simulink model "dimensions_equivalent"  (R2021b)
settings: Solver=VariableStepAuto  StartTime=0.0  StopTime=10.0  RelTol=1e-3
undefined symbols (not defined in the file): DiscIntNeverNeededParam, magnitude, Newton, Raphson
libraries: simulink x80, slpidlib x2
(part 1 of 3)
settings Model: Creator=user  LastModifiedBy=cemery
settings SolverCC: AlgebraicLoopSolver=TrustRegion
settings DataIOCC: ReturnWorkspaceOutputs=off
settings DebuggingCC: SFMachineParentedDataDiag=warning  ArithmeticOperatorsInVariantConditions=warning
settings SFSimCC: SimUseLocalCustomCode=off  CustomCodeUndefinedFunction=UseInterfaceOnly
settings RTWCC: RTWUseLocalCustomCode=off

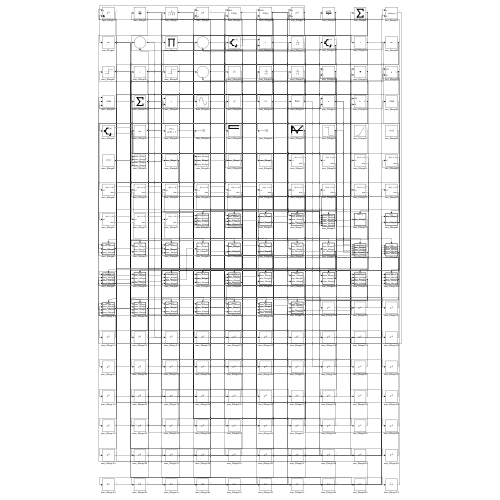
[thumbnail: Simulink's stored preview of the top-level diagram]
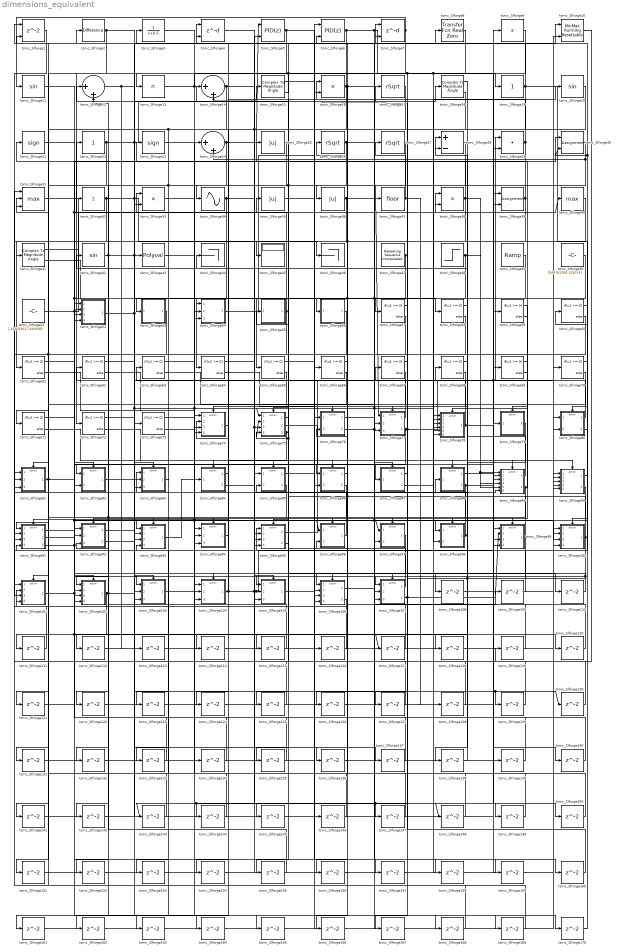
== system dimensions_equivalent ==
  tsmc_Slforge1 : Delay  ShowEnablePort=on  SampleTime=1
      settings: InputPortMap=u0,e6
  tsmc_Slforge10 : simulink/Math Operations/MinMax Running Resettable  Function=min  vinit=0.0
  tsmc_Slforge100 : Subsystem  TreatAsAtomicUnit=on
  tsmc_Slforge101 : Subsystem  TreatAsAtomicUnit=on
  tsmc_Slforge102 : Subsystem  TreatAsAtomicUnit=on
  tsmc_Slforge103 : Subsystem  TreatAsAtomicUnit=on
  tsmc_Slforge104 : Subsystem  TreatAsAtomicUnit=on
  tsmc_Slforge105 : Subsystem  TreatAsAtomicUnit=on
  tsmc_Slforge106 : Subsystem  TreatAsAtomicUnit=on
  tsmc_Slforge107 : Subsystem  TreatAsAtomicUnit=on
  tsmc_Slforge{108..170} (63 alike) : Delay  SampleTime=1
  tsmc_Slforge11 : Trigonometry
  tsmc_Slforge12 : Sum  Inputs=|++
  tsmc_Slforge13 : Product  Inputs=*
  tsmc_Slforge14 : Sum  Inputs=|++
  tsmc_Slforge15 : ComplexToMagnitudeAngle
  tsmc_Slforge16 : Product  Inputs=**
  tsmc_Slforge17 : Sqrt  Operator=rSqrt  AlgorithmType=Newton-Raphson  SaturateOnIntegerOverflow=on
  tsmc_Slforge18 : ComplexToMagnitudeAngle
  tsmc_Slforge19 : simulink/Math Operations/Slider Gain  gain=1  low=0  high=2
  tsmc_Slforge2 : simulink/Discrete/Difference  ICPrevInput=0.0  OutMin=[]  OutMax=[]  OutDataTypeStr=Inherit: Inherit via back propagation  OutDataType=fixdt(1, 16)  OutScaling=2^-10  DoSatur=off
  tsmc_Slforge20 : Trigonometry
  tsmc_Slforge21 : Signum
  tsmc_Slforge22 : simulink/Math Operations/Slider Gain  gain=1  low=0  high=2
  tsmc_Slforge23 : Signum
  tsmc_Slforge24 : Sum  Inputs=|++
  tsmc_Slforge25 : Abs
  tsmc_Slforge26 : Sqrt  Operator=rSqrt  AlgorithmType=Newton-Raphson  SaturateOnIntegerOverflow=on
  tsmc_Slforge27 : Sqrt  Operator=rSqrt  AlgorithmType=Newton-Raphson  SaturateOnIntegerOverflow=on
  tsmc_Slforge28 : Sum  Inputs=+-
  tsmc_Slforge29 : DotProduct  InputSameDT=on  OutDataTypeStr=Inherit: Inherit via internal rule
  tsmc_Slforge3 : DiscreteTransferFcn  SampleTime=1
  tsmc_Slforge30 : Assignment  DiagnosticForDimensions=Warning  IndexOptions=Index vector (dialog)  Indices=1  OutputSizes=1
  tsmc_Slforge31 : MinMax  Function=max  Inputs=3
  tsmc_Slforge32 : Sum  Inputs=+
  tsmc_Slforge33 : Product  Inputs=**
  tsmc_Slforge34 : Sin  TimeSource=Use external signal  SampleTime=0
  tsmc_Slforge35 : Abs
  tsmc_Slforge36 : Abs
  tsmc_Slforge37 : Rounding
  tsmc_Slforge38 : Product
  tsmc_Slforge39 : Assignment  DiagnosticForDimensions=Warning  IndexOptions=Index vector (dialog)  Indices=1  OutputSizes=1
  tsmc_Slforge4 : Delay  DelayLengthSource=Input port  SampleTime=1
      settings: InputPortMap=u0,p1
  tsmc_Slforge40 : MinMax  Function=max
  tsmc_Slforge41 : ComplexToMagnitudeAngle
  tsmc_Slforge42 : Trigonometry
  tsmc_Slforge43 : Polyval  Coefs=[ +2.081618890e-019, -1.441693666e-014, +4.719686976e-010, -8.536869453e-006, +1.621573104e-001, -8.087801117e+001 ]
  tsmc_Slforge44 : Terminator
  tsmc_Slforge45 : Display
  tsmc_Slforge46 : Terminator
  tsmc_Slforge47 : simulink/Sources/Repeating Sequence Interpolated  OutValues=[-224844362.242719, 761907502.904714, -469417062.555968, 95128126.771430, 892289046.180384]  TimeValues=[0 0.1 0.5 0.6 1].'  LookUpMeth=Use Input Below  tsamp=0.01  OutMin=[]  OutMax=[]  OutDataTypeStr=double  OutputDataTypeScalingMode=double  OutDataType=fixdt(0,8)  OutScaling=2^-10
  tsmc_Slforge48 : Step  Time=[25.000000]  Before=[335295422.757427]  After=[-716731590.646786]  SampleTime=0
  tsmc_Slforge49 : simulink/Sources/Ramp  slope=[-2914.888673]  start=[19.513339]  InitialOutput=[436099.857088]
  tsmc_Slforge5 : slpidlib/PID Controller (2DOF)  Controller=PID  Form=Parallel  TimeDomain=Discrete-time  UseExternalTs=off  SampleTime=1  IntegratorMethod=Forward Euler  FilterMethod=Forward Euler  ControllerParametersSource=internal  P=1  I=1  D=0  UseFilter=on  N=100  b=1  c=1  TunerSelectOption=Transfer Function Based (PID Tuner App)  InitialConditionSource=internal  InitialConditionForIntegrator=0  InitialConditionForFilter=0  DifferentiatorICPrevScaledInput=0  ExternalReset=none  TrackingMode=off  Kt=1  LimitOutput=off  SatLimitsSource=internal  UpperSaturationLimit=inf  LowerSaturationLimit=-inf  LinearizeAsGain=off  AntiWindupMode=none  Kb=1  POutMin=[]  POutMax=[]  IOutMin=[]  IOutMax=[]  DOutMin=[]  DOutMax=[]  NOutMin=[]  NOutMax=[]  bOutMin=[]  bOutMax=[]  cOutMin=[]  cOutMax=[]  SumOutMin=[]  SumOutMax=[]  SaturationOutMin=[]  SaturationOutMax=[]  PParamMin=[]  PParamMax=[]  IParamMin=[]  IParamMax=[]  DParamMin=[]  DParamMax=[]  NParamMin=[]  NParamMax=[]  bParamMin=[]  bParamMax=[]  cParamMin=[]  cParamMax=[]  KbParamMin=[]  KbParamMax=[]  KtParamMin=[]  KtParamMax=[]  KbOutMin=[]  KbOutMax=[]  KtOutMin=[]  KtOutMax=[]  IntegratorOutMin=[]  IntegratorOutMax=[]  FilterOutMin=[]  FilterOutMax=[]  SumI1OutMin=[]  SumI1OutMax=[]  SumI2OutMin=[]  SumI2OutMax=[]  SumI3OutMin=[]  SumI3OutMax=[]  SumI4OutMin=[]  SumI4OutMax=[]  SumDOutMin=[]  SumDOutMax=[]  Sum1OutMin=[]  Sum1OutMax=[]  Sum2OutMin=[]  Sum2OutMax=[]  Sum3OutMin=[]  Sum3OutMax=[]  DifferentiatorOutMin=[]  DifferentiatorOutMax=[]  FilterDiffOutCoefMin=[]  FilterDiffOutCoefMax=[]  ReciprocalOutMin=[]  ReciprocalOutMax=[]  SumDenOutMin=[]  SumDenOutMax=[]  SumNumOutMin=[]  SumNumOutMax=[]  DivideOutMin=[]  DivideOutMax=[]  UdiffTsProdOutMin=[]  UdiffTsProdOutMax=[]  NTsProdOutMin=[]  NTsProdOutMax=[]  UintegralTsProdOutMin=[]  UintegralTsProdOutMax=[]  UngainTsProdOutMin=[]  UngainTsProdOutMax=[]  IntegratorContinuousStateAttributes=''  IntegratorStateMustResolveToSignalObject=off  IntegratorRTWStateStorageClass=Auto  FilterContinuousStateAttributes=''  FilterStateMustResolveToSignalObject=off  FilterRTWStateStorageClass=Auto  ParallelPVariant=InternalParameters  IdealPVariant=Disabled  IVariant=InternalParameters  DVariant=InternalParameters  bVariant=InternalParameters  cVariant=InternalParameters  IntegratorVariant=Discrete  SatVariant=Disabled  AWVariant=Passthrough  PCopyVariant=Disabled  TRVariant=Disabled  FdbkBlocksVariant=Forward  IdealPFdbkVariant=Disabled  SatFdbkVariant=Disabled  DerivativeFilterVariant=ForwardEulerFilter  NVariant=InternalParameters  NCopyVariant=Disabled  FilterICVariant=InternalICsFilter  IntegratorICVariant=InternalICs  ExternalResetVariant=Disabled  TRSumVariant=Passthrough  SumFdbkVariant=Disabled  SumVariant=Sum_PID  TsampFilterVariant=InternalTs  TsampNgainVariant=Passthrough  TsampIntegralVariant=Passthrough  ExternalSaturationOutDataTypeStr=Inherit: Same as second input
      settings: SourceProductBaseCode=SL
  tsmc_Slforge50 : Constant  Value=[844181906.319014]  SampleTime=1
  tsmc_Slforge51 : Constant  Value=[-323053627.840698]  SampleTime=1
  tsmc_Slforge52 : Subsystem
  tsmc_Slforge53 : Subsystem
  tsmc_Slforge54 : Subsystem
  tsmc_Slforge55 : Subsystem
  tsmc_Slforge56 : Subsystem
  tsmc_Slforge{57..73} (17 alike) : If  IfExpression=u1 >= 0  SampleTime=1
  tsmc_Slforge6 : slpidlib/PID Controller (2DOF)  Controller=PID  Form=Parallel  TimeDomain=Discrete-time  UseExternalTs=off  SampleTime=1  IntegratorMethod=Forward Euler  FilterMethod=Forward Euler  ControllerParametersSource=internal  P=1  I=1  D=0  UseFilter=on  N=100  b=1  c=1  TunerSelectOption=Transfer Function Based (PID Tuner App)  InitialConditionSource=internal  InitialConditionForIntegrator=0  InitialConditionForFilter=0  DifferentiatorICPrevScaledInput=0  ExternalReset=none  TrackingMode=off  Kt=1  LimitOutput=off  SatLimitsSource=internal  UpperSaturationLimit=inf  LowerSaturationLimit=-inf  LinearizeAsGain=off  AntiWindupMode=none  Kb=1  POutMin=[]  POutMax=[]  IOutMin=[]  IOutMax=[]  DOutMin=[]  DOutMax=[]  NOutMin=[]  NOutMax=[]  bOutMin=[]  bOutMax=[]  cOutMin=[]  cOutMax=[]  SumOutMin=[]  SumOutMax=[]  SaturationOutMin=[]  SaturationOutMax=[]  PParamMin=[]  PParamMax=[]  IParamMin=[]  IParamMax=[]  DParamMin=[]  DParamMax=[]  NParamMin=[]  NParamMax=[]  bParamMin=[]  bParamMax=[]  cParamMin=[]  cParamMax=[]  KbParamMin=[]  KbParamMax=[]  KtParamMin=[]  KtParamMax=[]  KbOutMin=[]  KbOutMax=[]  KtOutMin=[]  KtOutMax=[]  IntegratorOutMin=[]  IntegratorOutMax=[]  FilterOutMin=[]  FilterOutMax=[]  SumI1OutMin=[]  SumI1OutMax=[]  SumI2OutMin=[]  SumI2OutMax=[]  SumI3OutMin=[]  SumI3OutMax=[]  SumI4OutMin=[]  SumI4OutMax=[]  SumDOutMin=[]  SumDOutMax=[]  Sum1OutMin=[]  Sum1OutMax=[]  Sum2OutMin=[]  Sum2OutMax=[]  Sum3OutMin=[]  Sum3OutMax=[]  DifferentiatorOutMin=[]  DifferentiatorOutMax=[]  FilterDiffOutCoefMin=[]  FilterDiffOutCoefMax=[]  ReciprocalOutMin=[]  ReciprocalOutMax=[]  SumDenOutMin=[]  SumDenOutMax=[]  SumNumOutMin=[]  SumNumOutMax=[]  DivideOutMin=[]  DivideOutMax=[]  UdiffTsProdOutMin=[]  UdiffTsProdOutMax=[]  NTsProdOutMin=[]  NTsProdOutMax=[]  UintegralTsProdOutMin=[]  UintegralTsProdOutMax=[]  UngainTsProdOutMin=[]  UngainTsProdOutMax=[]  IntegratorContinuousStateAttributes=''  IntegratorStateMustResolveToSignalObject=off  IntegratorRTWStateStorageClass=Auto  FilterContinuousStateAttributes=''  FilterStateMustResolveToSignalObject=off  FilterRTWStateStorageClass=Auto  ParallelPVariant=InternalParameters  IdealPVariant=Disabled  IVariant=InternalParameters  DVariant=InternalParameters  bVariant=InternalParameters  cVariant=InternalParameters  IntegratorVariant=Discrete  SatVariant=Disabled  AWVariant=Passthrough  PCopyVariant=Disabled  TRVariant=Disabled  FdbkBlocksVariant=Forward  IdealPFdbkVariant=Disabled  SatFdbkVariant=Disabled  DerivativeFilterVariant=ForwardEulerFilter  NVariant=InternalParameters  NCopyVariant=Disabled  FilterICVariant=InternalICsFilter  IntegratorICVariant=InternalICs  ExternalResetVariant=Disabled  TRSumVariant=Passthrough  SumFdbkVariant=Disabled  SumVariant=Sum_PID  TsampFilterVariant=InternalTs  TsampNgainVariant=Passthrough  TsampIntegralVariant=Passthrough  ExternalSaturationOutDataTypeStr=Inherit: Same as second input
      settings: SourceProductBaseCode=SL
  tsmc_Slforge7 : Delay  DelayLengthSource=Input port  SampleTime=1
      settings: InputPortMap=u0,p1
  tsmc_Slforge74 : Subsystem  TreatAsAtomicUnit=on
  tsmc_Slforge75 : Subsystem  TreatAsAtomicUnit=on
  tsmc_Slforge76 : Subsystem  TreatAsAtomicUnit=on
  tsmc_Slforge77 : Subsystem  TreatAsAtomicUnit=on
  tsmc_Slforge78 : Subsystem  TreatAsAtomicUnit=on
  tsmc_Slforge79 : Subsystem  TreatAsAtomicUnit=on
  tsmc_Slforge8 : simulink/Discrete/Transfer Fcn Real Zero  ZeroZ=0.75  ICPrevInput=0.0  DoSatur=off
      settings: SourceProductBaseCode=SL
  tsmc_Slforge80 : Subsystem  TreatAsAtomicUnit=on
  tsmc_Slforge81 : Subsystem  TreatAsAtomicUnit=on
  tsmc_Slforge82 : Subsystem  TreatAsAtomicUnit=on
  tsmc_Slforge83 : Subsystem  TreatAsAtomicUnit=on
  tsmc_Slforge84 : Subsystem  TreatAsAtomicUnit=on
  tsmc_Slforge85 : Subsystem  TreatAsAtomicUnit=on
  tsmc_Slforge86 : Subsystem  TreatAsAtomicUnit=on
  tsmc_Slforge87 : Subsystem  TreatAsAtomicUnit=on
  tsmc_Slforge88 : Subsystem  TreatAsAtomicUnit=on
  tsmc_Slforge89 : Subsystem  TreatAsAtomicUnit=on
  tsmc_Slforge9 : Sum  Inputs=+
  tsmc_Slforge90 : Subsystem  TreatAsAtomicUnit=on
  tsmc_Slforge91 : Subsystem  TreatAsAtomicUnit=on
  tsmc_Slforge92 : Subsystem  TreatAsAtomicUnit=on
  tsmc_Slforge93 : Subsystem  TreatAsAtomicUnit=on
  tsmc_Slforge94 : Subsystem  TreatAsAtomicUnit=on
  tsmc_Slforge95 : Subsystem  TreatAsAtomicUnit=on
  tsmc_Slforge96 : Subsystem  TreatAsAtomicUnit=on
  tsmc_Slforge97 : Subsystem  TreatAsAtomicUnit=on
  tsmc_Slforge98 : Subsystem  TreatAsAtomicUnit=on
  tsmc_Slforge99 : Subsystem  TreatAsAtomicUnit=on
  wires:
  tsmc_Slforge26/1 -> tsmc_Slforge162/1, tsmc_Slforge163/1, tsmc_Slforge89/3(tsmc_Slforge25)
  tsmc_Slforge95/1(tsmc_Slforge2) -> tsmc_Slforge29/1
  tsmc_Slforge36/1 -> tsmc_Slforge77/1(tsmc_Slforge1), tsmc_Slforge45/1
  tsmc_Slforge102/1(tsmc_Slforge2) -> tsmc_Slforge129/1, tsmc_Slforge130/1, tsmc_Slforge132/1, tsmc_Slforge131/1
  tsmc_Slforge50/1 -> tsmc_Slforge53/1(tsmc_Slforge1)
  tsmc_Slforge49/1 -> tsmc_Slforge64/1
  tsmc_Slforge19/1 -> tsmc_Slforge95/1(tsmc_Slforge1), tsmc_Slforge7/2, tsmc_Slforge95/4(tsmc_Slforge28)
  tsmc_Slforge93/1(tsmc_Slforge2) -> tsmc_Slforge84/1(tsmc_Slforge1)
  tsmc_Slforge39/1 -> tsmc_Slforge102/4(tsmc_Slforge29), tsmc_Slforge156/1, tsmc_Slforge36/1
  tsmc_Slforge2/1 -> tsmc_Slforge95/2(tsmc_Slforge26), tsmc_Slforge78/6(tsmc_Slforge24), tsmc_Slforge72/1
  tsmc_Slforge32/1 -> tsmc_Slforge46/1, tsmc_Slforge169/1, tsmc_Slforge101/3(tsmc_Slforge30)
  tsmc_Slforge3/1 -> tsmc_Slforge147/1, tsmc_Slforge148/1
  tsmc_Slforge51/1 -> tsmc_Slforge33/1, tsmc_Slforge89/2(tsmc_Slforge24)
  tsmc_Slforge100/1(tsmc_Slforge2) -> tsmc_Slforge103/3(tsmc_Slforge27), tsmc_Slforge167/1, tsmc_Slforge16/1, tsmc_Slforge75/4(tsmc_Slforge29)
  tsmc_Slforge55/1(tsmc_Slforge2) -> tsmc_Slforge22/1, tsmc_Slforge82/2(tsmc_Slforge24)
  tsmc_Slforge16/1 -> tsmc_Slforge78/2(tsmc_Slforge20), tsmc_Slforge166/1, tsmc_Slforge13/1, tsmc_Slforge102/3(tsmc_Slforge28)
  tsmc_Slforge40/1 -> tsmc_Slforge61/1
  tsmc_Slforge37/1 -> tsmc_Slforge27/1, tsmc_Slforge128/1
  tsmc_Slforge27/1 -> tsmc_Slforge33/2
  tsmc_Slforge8/1 -> tsmc_Slforge37/1, tsmc_Slforge98/2(tsmc_Slforge29)
  tsmc_Slforge99/1(tsmc_Slforge2) -> tsmc_Slforge143/1, tsmc_Slforge144/1, tsmc_Slforge138/1, tsmc_Slforge28/1
  tsmc_Slforge98/1(tsmc_Slforge2) -> tsmc_Slforge14/1, tsmc_Slforge28/2
  tsmc_Slforge22/1 -> tsmc_Slforge75/1(tsmc_Slforge1), tsmc_Slforge74/4(tsmc_Slforge25), tsmc_Slforge17/1, tsmc_Slforge32/1
  tsmc_Slforge7/1 -> tsmc_Slforge105/1(tsmc_Slforge1), tsmc_Slforge74/3(tsmc_Slforge24), tsmc_Slforge11/1
  tsmc_Slforge9/1 -> tsmc_Slforge41/1, tsmc_Slforge57/1
  tsmc_Slforge34/1 -> tsmc_Slforge54/1(tsmc_Slforge1), tsmc_Slforge58/1
  tsmc_Slforge78/1(tsmc_Slforge2) -> tsmc_Slforge4/1, tsmc_Slforge150/1
  tsmc_Slforge30/1 -> tsmc_Slforge24/2, tsmc_Slforge103/2(tsmc_Slforge26)
  tsmc_Slforge53/1(tsmc_Slforge2) -> tsmc_Slforge91/1(tsmc_Slforge1), tsmc_Slforge81/3(tsmc_Slforge25)
  tsmc_Slforge24/1 -> tsmc_Slforge5/1, tsmc_Slforge71/1
  tsmc_Slforge95/2(tsmc_Slforge29) -> tsmc_Slforge63/1, tsmc_Slforge75/2(tsmc_Slforge27)
  tsmc_Slforge76/1(tsmc_Slforge2) -> tsmc_Slforge8/1
  tsmc_Slforge17/1 -> tsmc_Slforge106/2(tsmc_Slforge19)
  tsmc_Slforge13/1 -> tsmc_Slforge78/4(tsmc_Slforge22), tsmc_Slforge165/1, tsmc_Slforge19/1
  tsmc_Slforge35/1 -> tsmc_Slforge10/1
  tsmc_Slforge28/1 -> tsmc_Slforge102/1(tsmc_Slforge1), tsmc_Slforge133/1
  tsmc_Slforge11/1 -> tsmc_Slforge117/1, tsmc_Slforge160/1, tsmc_Slforge54/3(tsmc_Slforge11)
  tsmc_Slforge41/1 -> tsmc_Slforge56/1(tsmc_Slforge1)
  tsmc_Slforge84/1(tsmc_Slforge2) -> tsmc_Slforge94/3(tsmc_Slforge31)
  tsmc_Slforge31/1 -> tsmc_Slforge65/1
  tsmc_Slforge75/2(tsmc_Slforge30) -> tsmc_Slforge87/1(tsmc_Slforge1)
  tsmc_Slforge52/1(tsmc_Slforge2) -> tsmc_Slforge18/1, tsmc_Slforge99/4(tsmc_Slforge28)
  tsmc_Slforge107/1(tsmc_Slforge2) -> tsmc_Slforge12/1
  tsmc_Slforge23/1 -> tsmc_Slforge96/1(tsmc_Slforge1), tsmc_Slforge145/1
  tsmc_Slforge90/1(tsmc_Slforge2) -> tsmc_Slforge93/1(tsmc_Slforge1)
  tsmc_Slforge29/1 -> tsmc_Slforge114/1, tsmc_Slforge115/1, tsmc_Slforge4/2
  tsmc_Slforge48/1 -> tsmc_Slforge77/2(tsmc_Slforge29), tsmc_Slforge93/3(tsmc_Slforge22), tsmc_Slforge89/5(tsmc_Slforge27)
  tsmc_Slforge1/1 -> tsmc_Slforge81/2(tsmc_Slforge24)
  tsmc_Slforge21/1 -> tsmc_Slforge103/1(tsmc_Slforge1), tsmc_Slforge97/1(tsmc_Slforge1)
  tsmc_Slforge107/2(tsmc_Slforge28) -> tsmc_Slforge83/1(tsmc_Slforge1), tsmc_Slforge99/2(tsmc_Slforge26)
  tsmc_Slforge47/1 -> tsmc_Slforge86/1(tsmc_Slforge1), tsmc_Slforge86/2(tsmc_Slforge28), tsmc_Slforge107/1(tsmc_Slforge1)
  tsmc_Slforge5/1 -> tsmc_Slforge104/3(tsmc_Slforge28), tsmc_Slforge157/1
  tsmc_Slforge12/1 -> tsmc_Slforge100/3(tsmc_Slforge26), tsmc_Slforge113/1
  tsmc_Slforge20/1 -> tsmc_Slforge83/3(tsmc_Slforge29), tsmc_Slforge153/1
  tsmc_Slforge14/1 -> tsmc_Slforge120/1, tsmc_Slforge121/1
  tsmc_Slforge91/2(tsmc_Slforge25) -> tsmc_Slforge25/1
  tsmc_Slforge54/1(tsmc_Slforge2) -> tsmc_Slforge6/1
  tsmc_Slforge96/1(tsmc_Slforge2) -> tsmc_Slforge15/1
  tsmc_Slforge88/2(tsmc_Slforge30) -> tsmc_Slforge141/1, tsmc_Slforge142/1, tsmc_Slforge140/1
  tsmc_Slforge87/2(tsmc_Slforge24) -> tsmc_Slforge20/1
  tsmc_Slforge81/1(tsmc_Slforge2) -> tsmc_Slforge31/2, tsmc_Slforge170/1
  tsmc_Slforge104/1(tsmc_Slforge2) -> tsmc_Slforge39/2, tsmc_Slforge105/2(tsmc_Slforge24), tsmc_Slforge89/6(tsmc_Slforge28), tsmc_Slforge74/2(tsmc_Slforge23)
  tsmc_Slforge91/3(tsmc_Slforge26) -> tsmc_Slforge52/2(tsmc_Slforge8), tsmc_Slforge168/1
  tsmc_Slforge15/2 -> tsmc_Slforge3/1
  tsmc_Slforge80/1(tsmc_Slforge2) -> tsmc_Slforge55/1(tsmc_Slforge1)
  tsmc_Slforge106/2(tsmc_Slforge22) -> tsmc_Slforge101/2(tsmc_Slforge29)
  tsmc_Slforge101/1(tsmc_Slforge2) -> tsmc_Slforge30/1, tsmc_Slforge40/1, tsmc_Slforge158/1
  tsmc_Slforge6/1 -> tsmc_Slforge105/3(tsmc_Slforge25), tsmc_Slforge75/3(tsmc_Slforge28), tsmc_Slforge78/3(tsmc_Slforge21), tsmc_Slforge159/1, tsmc_Slforge79/1(tsmc_Slforge1)
  tsmc_Slforge90/2(tsmc_Slforge27) -> tsmc_Slforge92/2(tsmc_Slforge29), tsmc_Slforge97/2(tsmc_Slforge25)
  tsmc_Slforge41/2 -> tsmc_Slforge83/2(tsmc_Slforge28)
  tsmc_Slforge77/1(tsmc_Slforge2) -> tsmc_Slforge35/1
  tsmc_Slforge94/1(tsmc_Slforge2) -> tsmc_Slforge44/1
  tsmc_Slforge105/1(tsmc_Slforge2) -> tsmc_Slforge38/1
  tsmc_Slforge18/2 -> tsmc_Slforge34/1, tsmc_Slforge95/3(tsmc_Slforge27)
  tsmc_Slforge42/1 -> tsmc_Slforge43/1, tsmc_Slforge99/3(tsmc_Slforge27), tsmc_Slforge82/1(tsmc_Slforge1)
  tsmc_Slforge77/2(tsmc_Slforge31) -> tsmc_Slforge10/2, tsmc_Slforge9/1, tsmc_Slforge14/2, tsmc_Slforge102/2(tsmc_Slforge27)
  tsmc_Slforge38/1 -> tsmc_Slforge89/1(tsmc_Slforge1), tsmc_Slforge89/4(tsmc_Slforge26), tsmc_Slforge21/1, tsmc_Slforge152/1
  tsmc_Slforge92/1(tsmc_Slforge2) -> tsmc_Slforge7/1
  tsmc_Slforge89/1(tsmc_Slforge2) -> tsmc_Slforge42/1
  tsmc_Slforge80/2(tsmc_Slforge22) -> tsmc_Slforge2/1, tsmc_Slforge30/2
  tsmc_Slforge75/3(tsmc_Slforge31) -> tsmc_Slforge154/1, tsmc_Slforge155/1
  tsmc_Slforge86/1(tsmc_Slforge2) -> tsmc_Slforge26/1
  tsmc_Slforge89/2(tsmc_Slforge29) -> tsmc_Slforge23/1, tsmc_Slforge151/1
  tsmc_Slforge76/2(tsmc_Slforge24) -> tsmc_Slforge38/2, tsmc_Slforge98/1(tsmc_Slforge1)
  tsmc_Slforge92/2(tsmc_Slforge31) -> tsmc_Slforge68/1
  tsmc_Slforge57/1 -> tsmc_Slforge74/Action
  tsmc_Slforge57/2 -> tsmc_Slforge75/Action
  tsmc_Slforge58/1 -> tsmc_Slforge76/Action
  tsmc_Slforge58/2 -> tsmc_Slforge77/Action
  tsmc_Slforge59/1 -> tsmc_Slforge78/Action
  tsmc_Slforge59/2 -> tsmc_Slforge79/Action
  tsmc_Slforge60/1 -> tsmc_Slforge80/Action
  tsmc_Slforge60/2 -> tsmc_Slforge81/Action
  tsmc_Slforge61/1 -> tsmc_Slforge82/Action
  tsmc_Slforge61/2 -> tsmc_Slforge83/Action
  tsmc_Slforge62/1 -> tsmc_Slforge84/Action
  tsmc_Slforge62/2 -> tsmc_Slforge85/Action
  tsmc_Slforge63/1 -> tsmc_Slforge86/Action
  tsmc_Slforge63/2 -> tsmc_Slforge87/Action
  tsmc_Slforge64/1 -> tsmc_Slforge88/Action
  tsmc_Slforge64/2 -> tsmc_Slforge89/Action
  tsmc_Slforge65/1 -> tsmc_Slforge90/Action
  tsmc_Slforge65/2 -> tsmc_Slforge91/Action
  tsmc_Slforge66/1 -> tsmc_Slforge92/Action
  tsmc_Slforge66/2 -> tsmc_Slforge93/Action
  tsmc_Slforge67/1 -> tsmc_Slforge94/Action
  tsmc_Slforge67/2 -> tsmc_Slforge95/Action
  tsmc_Slforge68/1 -> tsmc_Slforge96/Action
  tsmc_Slforge68/2 -> tsmc_Slforge97/Action
  tsmc_Slforge69/1 -> tsmc_Slforge98/Action
  tsmc_Slforge69/2 -> tsmc_Slforge99/Action
  tsmc_Slforge70/1 -> tsmc_Slforge100/Action
  tsmc_Slforge70/2 -> tsmc_Slforge101/Action
  tsmc_Slforge71/1 -> tsmc_Slforge102/Action
  tsmc_Slforge71/2 -> tsmc_Slforge103/Action
  tsmc_Slforge72/1 -> tsmc_Slforge104/Action
  tsmc_Slforge72/2 -> tsmc_Slforge105/Action
  tsmc_Slforge73/1 -> tsmc_Slforge106/Action
  tsmc_Slforge73/2 -> tsmc_Slforge107/Action
  tsmc_Slforge84/2(tsmc_Slforge27) -> tsmc_Slforge108/1
  tsmc_Slforge108/1 -> tsmc_Slforge80/1(tsmc_Slforge1)
  tsmc_Slforge106/1(tsmc_Slforge2) -> tsmc_Slforge109/1
  tsmc_Slforge109/1 -> tsmc_Slforge91/2(tsmc_Slforge22)
  tsmc_Slforge91/1(tsmc_Slforge2) -> tsmc_Slforge110/1
  tsmc_Slforge110/1 -> tsmc_Slforge106/1(tsmc_Slforge1)
  tsmc_Slforge25/1 -> tsmc_Slforge111/1
  tsmc_Slforge111/1 -> tsmc_Slforge31/1
  tsmc_Slforge18/1 -> tsmc_Slforge112/1
  tsmc_Slforge112/1 -> tsmc_Slforge73/1
  tsmc_Slforge113/1 -> tsmc_Slforge80/2(tsmc_Slforge21)
  tsmc_Slforge114/1 -> tsmc_Slforge16/2
  tsmc_Slforge115/1 -> tsmc_Slforge62/1
  tsmc_Slforge85/1(tsmc_Slforge2) -> tsmc_Slforge116/1
  tsmc_Slforge116/1 -> tsmc_Slforge92/1(tsmc_Slforge1)
  tsmc_Slforge117/1 -> tsmc_Slforge81/1(tsmc_Slforge1)
  tsmc_Slforge79/1(tsmc_Slforge2) -> tsmc_Slforge118/1
  tsmc_Slforge118/1 -> tsmc_Slforge70/1
  tsmc_Slforge10/1 -> tsmc_Slforge119/1
  tsmc_Slforge119/1 -> tsmc_Slforge94/1(tsmc_Slforge1)
  tsmc_Slforge120/1 -> tsmc_Slforge1/1
  tsmc_Slforge121/1 -> tsmc_Slforge52/4(tsmc_Slforge10)
  tsmc_Slforge56/1(tsmc_Slforge2) -> tsmc_Slforge122/1
  tsmc_Slforge122/1 -> tsmc_Slforge24/1
  tsmc_Slforge83/1(tsmc_Slforge2) -> tsmc_Slforge123/1
  tsmc_Slforge123/1 -> tsmc_Slforge77/3(tsmc_Slforge30)
  tsmc_Slforge74/1(tsmc_Slforge2) -> tsmc_Slforge124/1
  tsmc_Slforge124/1 -> tsmc_Slforge39/1
  tsmc_Slforge75/1(tsmc_Slforge2) -> tsmc_Slforge125/1
  tsmc_Slforge125/1 -> tsmc_Slforge104/2(tsmc_Slforge27)
  tsmc_Slforge87/1(tsmc_Slforge2) -> tsmc_Slforge126/1
  tsmc_Slforge126/1 -> tsmc_Slforge76/2(tsmc_Slforge23)
  tsmc_Slforge33/1 -> tsmc_Slforge127/1
  tsmc_Slforge127/1 -> tsmc_Slforge85/2(tsmc_Slforge21)
  tsmc_Slforge128/1 -> tsmc_Slforge101/4(tsmc_Slforge31)
  tsmc_Slforge129/1 -> tsmc_Slforge101/1(tsmc_Slforge1)
  tsmc_Slforge130/1 -> tsmc_Slforge92/3(tsmc_Slforge30)
  tsmc_Slforge131/1 -> tsmc_Slforge106/4(tsmc_Slforge21)
  tsmc_Slforge132/1 -> tsmc_Slforge54/2(tsmc_Slforge10)
  tsmc_Slforge133/1 -> tsmc_Slforge52/3(tsmc_Slforge9)
  tsmc_Slforge103/1(tsmc_Slforge2) -> tsmc_Slforge134/1
  tsmc_Slforge134/1 -> tsmc_Slforge104/1(tsmc_Slforge1)
  tsmc_Slforge97/1(tsmc_Slforge2) -> tsmc_Slforge135/1
  tsmc_Slforge135/1 -> tsmc_Slforge52/1(tsmc_Slforge1)
  tsmc_Slforge43/1 -> tsmc_Slforge136/1
  tsmc_Slforge136/1 -> tsmc_Slforge29/2
  tsmc_Slforge82/1(tsmc_Slforge2) -> tsmc_Slforge137/1
  tsmc_Slforge137/1 -> tsmc_Slforge6/2
  tsmc_Slforge138/1 -> tsmc_Slforge88/1(tsmc_Slforge1)
  tsmc_Slforge88/1(tsmc_Slforge2) -> tsmc_Slforge139/1
  tsmc_Slforge139/1 -> tsmc_Slforge85/1(tsmc_Slforge1)
  tsmc_Slforge140/1 -> tsmc_Slforge99/1(tsmc_Slforge1)
  tsmc_Slforge141/1 -> tsmc_Slforge69/1
  tsmc_Slforge142/1 -> tsmc_Slforge93/2(tsmc_Slforge21)
  tsmc_Slforge143/1 -> tsmc_Slforge91/4(tsmc_Slforge24)
  tsmc_Slforge144/1 -> tsmc_Slforge1/2
  tsmc_Slforge145/1 -> tsmc_Slforge106/3(tsmc_Slforge20)
  tsmc_Slforge15/1 -> tsmc_Slforge146/1
  tsmc_Slforge146/1 -> tsmc_Slforge76/1(tsmc_Slforge1)
  tsmc_Slforge147/1 -> tsmc_Slforge74/1(tsmc_Slforge1)
  tsmc_Slforge148/1 -> tsmc_Slforge96/2(tsmc_Slforge29)
  tsmc_Slforge4/1 -> tsmc_Slforge149/1
  tsmc_Slforge149/1 -> tsmc_Slforge94/2(tsmc_Slforge30)
  tsmc_Slforge150/1 -> tsmc_Slforge93/4(tsmc_Slforge23)
  tsmc_Slforge151/1 -> tsmc_Slforge59/1
  tsmc_Slforge152/1 -> tsmc_Slforge78/5(tsmc_Slforge23)
  tsmc_Slforge153/1 -> tsmc_Slforge5/2
  tsmc_Slforge154/1 -> tsmc_Slforge90/1(tsmc_Slforge1)
  tsmc_Slforge155/1 -> tsmc_Slforge12/2
  tsmc_Slforge156/1 -> tsmc_Slforge78/1(tsmc_Slforge1)
  tsmc_Slforge157/1 -> tsmc_Slforge100/4(tsmc_Slforge27)
  tsmc_Slforge158/1 -> tsmc_Slforge90/2(tsmc_Slforge23)
  tsmc_Slforge159/1 -> tsmc_Slforge90/4(tsmc_Slforge25)
  tsmc_Slforge160/1 -> tsmc_Slforge67/1
  tsmc_Slforge85/2(tsmc_Slforge22) -> tsmc_Slforge161/1
  tsmc_Slforge161/1 -> tsmc_Slforge100/1(tsmc_Slforge1)
  tsmc_Slforge162/1 -> tsmc_Slforge66/1
  tsmc_Slforge163/1 -> tsmc_Slforge107/2(tsmc_Slforge26)
  tsmc_Slforge86/2(tsmc_Slforge29) -> tsmc_Slforge164/1
  tsmc_Slforge164/1 -> tsmc_Slforge100/2(tsmc_Slforge25)
  tsmc_Slforge165/1 -> tsmc_Slforge107/3(tsmc_Slforge27)
  tsmc_Slforge166/1 -> tsmc_Slforge90/5(tsmc_Slforge26)
  tsmc_Slforge167/1 -> tsmc_Slforge90/3(tsmc_Slforge24)
  tsmc_Slforge168/1 -> tsmc_Slforge31/3
  tsmc_Slforge169/1 -> tsmc_Slforge91/3(tsmc_Slforge23)
  tsmc_Slforge170/1 -> tsmc_Slforge60/1

== system dimensions_equivalent/tsmc_Slforge100 ==
  tsmc_Slforge1 : Inport
  tsmc_Slforge25 : Inport  Port=2
  tsmc_Slforge26 : Inport  Port=3
  tsmc_Slforge27 : Inport  Port=4
  Action Port : ActionPort  ActionPortLabel=if { }
  tsmc_Slforge10 : Squeeze
  tsmc_Slforge11 : Math  Operator=magnitude^2  SignedPower=on  SaturateOnIntegerOverflow=on
  tsmc_Slforge12 : Sum  Inputs=+-
  tsmc_Slforge13 : Sum  Inputs=--
  tsmc_Slforge14 : Product
  tsmc_Slforge15 : Sum  Inputs=+-
  tsmc_Slforge16 : simulink/Math Operations/Slider Gain  gain=1  low=0  high=2
  tsmc_Slforge17 : Sqrt  Operator=rSqrt  AlgorithmType=Newton-Raphson  SaturateOnIntegerOverflow=on
  tsmc_Slforge18 : Sum  Inputs=|++
  tsmc_Slforge19 : Sum  Inputs=|++
  tsmc_Slforge20 : PermuteDimensions
  tsmc_Slforge21 : Bias  Bias=[40352577.982975]
  tsmc_Slforge22 : ComplexToRealImag
  tsmc_Slforge23 : UnaryMinus
  tsmc_Slforge24 : Polyval  Coefs=[ +2.081618890e-019, -1.441693666e-014, +4.719686976e-010, -8.536869453e-006, +1.621573104e-001, -8.087801117e+001 ]
  tsmc_Slforge28 : Delay
  tsmc_Slforge3 : Delay
  tsmc_Slforge4 : simulink/Discrete/Transfer Fcn Real Zero  ZeroZ=0.75  ICPrevInput=0.0  DoSatur=off
      settings: SourceProductBaseCode=SL
  tsmc_Slforge5 : simulink/Discrete/Transfer Fcn First Order  PoleZ=0.95  ICPrevOutput=0.0  DoSatur=off
  tsmc_Slforge6 : Math  Operator=pow  SignedPower=on  SaturateOnIntegerOverflow=on
  tsmc_Slforge7 : Squeeze
  tsmc_Slforge8 : Squeeze
  tsmc_Slforge9 : Gain  Gain=[571889699.729792]
  tsmc_Slforge2 : Outport  VectorParamsAs1DForOutWhenUnconnected=off
  wires:
  tsmc_Slforge24/1 -> tsmc_Slforge3/1
  tsmc_Slforge5/1 -> tsmc_Slforge4/1
  tsmc_Slforge9/1 -> tsmc_Slforge11/1, tsmc_Slforge19/2
  tsmc_Slforge7/1 -> tsmc_Slforge15/1
  tsmc_Slforge22/1 -> tsmc_Slforge15/2
  tsmc_Slforge10/1 -> tsmc_Slforge20/1
  tsmc_Slforge22/2 -> tsmc_Slforge14/1, tsmc_Slforge12/1
  tsmc_Slforge26/1 -> tsmc_Slforge16/1
  tsmc_Slforge8/1 -> tsmc_Slforge21/1
  tsmc_Slforge25/1 -> tsmc_Slforge14/2
  tsmc_Slforge6/1 -> tsmc_Slforge22/1, tsmc_Slforge12/2
  tsmc_Slforge13/1 -> tsmc_Slforge17/1
  tsmc_Slforge14/1 -> tsmc_Slforge7/1
  tsmc_Slforge21/1 -> tsmc_Slforge24/1
  tsmc_Slforge20/1 -> tsmc_Slforge6/1
  tsmc_Slforge16/1 -> tsmc_Slforge8/1
  tsmc_Slforge23/1 -> tsmc_Slforge13/1
  tsmc_Slforge19/1 -> tsmc_Slforge2/1
  tsmc_Slforge27/1 -> tsmc_Slforge13/2
  tsmc_Slforge15/1 -> tsmc_Slforge18/2
  tsmc_Slforge12/1 -> tsmc_Slforge19/1
  tsmc_Slforge3/1 -> tsmc_Slforge23/1
  tsmc_Slforge1/1 -> tsmc_Slforge5/1
  tsmc_Slforge4/1 -> tsmc_Slforge10/1
  tsmc_Slforge17/1 -> tsmc_Slforge6/2
  tsmc_Slforge18/1 -> tsmc_Slforge9/1
  tsmc_Slforge11/1 -> tsmc_Slforge28/1
  tsmc_Slforge28/1 -> tsmc_Slforge18/1

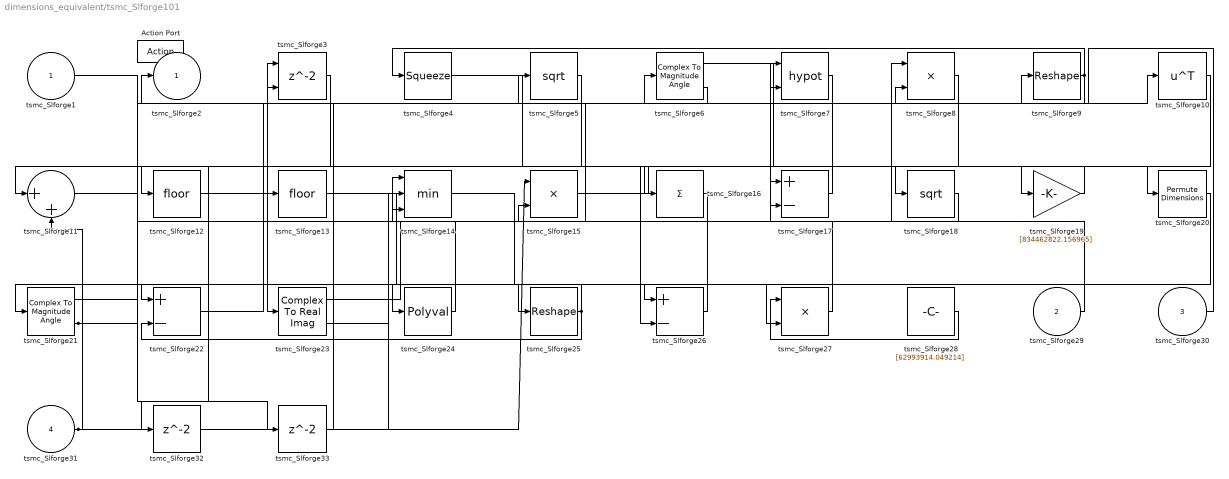
== system dimensions_equivalent/tsmc_Slforge101 ==
  tsmc_Slforge1 : Inport
  tsmc_Slforge29 : Inport  Port=2
  tsmc_Slforge30 : Inport  Port=3
  tsmc_Slforge31 : Inport  Port=4
  Action Port : ActionPort  ActionPortLabel=else { }
  tsmc_Slforge10 : Math  Operator=transpose  SignedPower=on  SaturateOnIntegerOverflow=on
  tsmc_Slforge11 : Sum  Inputs=|++
  tsmc_Slforge12 : Rounding
  tsmc_Slforge13 : Rounding
  tsmc_Slforge14 : MinMax  Inputs=3
  tsmc_Slforge15 : Product
  tsmc_Slforge16 : Sum  Inputs=+
  tsmc_Slforge17 : Sum  Inputs=+-
  tsmc_Slforge18 : Sqrt  SaturateOnIntegerOverflow=on
  tsmc_Slforge19 : Gain  Gain=[834462822.156965]
  tsmc_Slforge20 : PermuteDimensions
  tsmc_Slforge21 : ComplexToMagnitudeAngle
  tsmc_Slforge22 : Sum  Inputs=+-
  tsmc_Slforge23 : ComplexToRealImag
  tsmc_Slforge24 : Polyval  Coefs=[ +2.081618890e-019, -1.441693666e-014, +4.719686976e-010, -8.536869453e-006, +1.621573104e-001, -8.087801117e+001 ]
  tsmc_Slforge25 : Reshape
  tsmc_Slforge26 : Sum  Inputs=+-
  tsmc_Slforge27 : Product  Inputs=**
  tsmc_Slforge28 : Constant  Value=[62993914.049214]  SampleTime=1
  tsmc_Slforge3 : Delay  ShowEnablePort=on
      settings: InputPortMap=u0,e6
  tsmc_Slforge32 : Delay
  tsmc_Slforge33 : Delay
  tsmc_Slforge4 : Squeeze
  tsmc_Slforge5 : Sqrt  SaturateOnIntegerOverflow=on
  tsmc_Slforge6 : ComplexToMagnitudeAngle
  tsmc_Slforge7 : Math  Operator=hypot  SignedPower=on  SaturateOnIntegerOverflow=on
  tsmc_Slforge8 : Product
  tsmc_Slforge9 : Reshape
  tsmc_Slforge2 : Outport  VectorParamsAs1DForOutWhenUnconnected=off
  wires:
  tsmc_Slforge5/1 -> tsmc_Slforge12/1
  tsmc_Slforge31/1 -> tsmc_Slforge15/1, tsmc_Slforge11/2
  tsmc_Slforge6/1 -> tsmc_Slforge19/1
  tsmc_Slforge9/1 -> tsmc_Slforge4/1, tsmc_Slforge8/2
  tsmc_Slforge20/1 -> tsmc_Slforge26/1
  tsmc_Slforge28/1 -> tsmc_Slforge27/1
  tsmc_Slforge18/1 -> tsmc_Slforge7/1
  tsmc_Slforge16/1 -> tsmc_Slforge22/1
  tsmc_Slforge8/1 -> tsmc_Slforge26/2
  tsmc_Slforge6/2 -> tsmc_Slforge2/1
  tsmc_Slforge25/1 -> tsmc_Slforge21/1, tsmc_Slforge22/2
  tsmc_Slforge15/1 -> tsmc_Slforge18/1
  tsmc_Slforge12/1 -> tsmc_Slforge3/1
  tsmc_Slforge10/1 -> tsmc_Slforge23/1
  tsmc_Slforge4/1 -> tsmc_Slforge20/1
  tsmc_Slforge13/1 -> tsmc_Slforge25/1
  tsmc_Slforge19/1 -> tsmc_Slforge16/1
  tsmc_Slforge21/1 -> tsmc_Slforge15/2
  tsmc_Slforge17/1 -> tsmc_Slforge11/1
  tsmc_Slforge21/2 -> tsmc_Slforge7/2, tsmc_Slforge33/1
  tsmc_Slforge27/1 -> tsmc_Slforge5/1
  tsmc_Slforge30/1 -> tsmc_Slforge9/1
  tsmc_Slforge24/1 -> tsmc_Slforge3/2
  tsmc_Slforge7/1 -> tsmc_Slforge17/1
  tsmc_Slforge23/1 -> tsmc_Slforge8/1
  tsmc_Slforge22/1 -> tsmc_Slforge10/1
  tsmc_Slforge11/1 -> tsmc_Slforge24/1
  tsmc_Slforge1/1 -> tsmc_Slforge6/1
  tsmc_Slforge23/2 -> tsmc_Slforge17/2
  tsmc_Slforge29/1 -> tsmc_Slforge14/1
  tsmc_Slforge26/1 -> tsmc_Slforge14/3
  tsmc_Slforge14/1 -> tsmc_Slforge27/2
  tsmc_Slforge3/1 -> tsmc_Slforge32/1
  tsmc_Slforge32/1 -> tsmc_Slforge14/2
  tsmc_Slforge33/1 -> tsmc_Slforge13/1

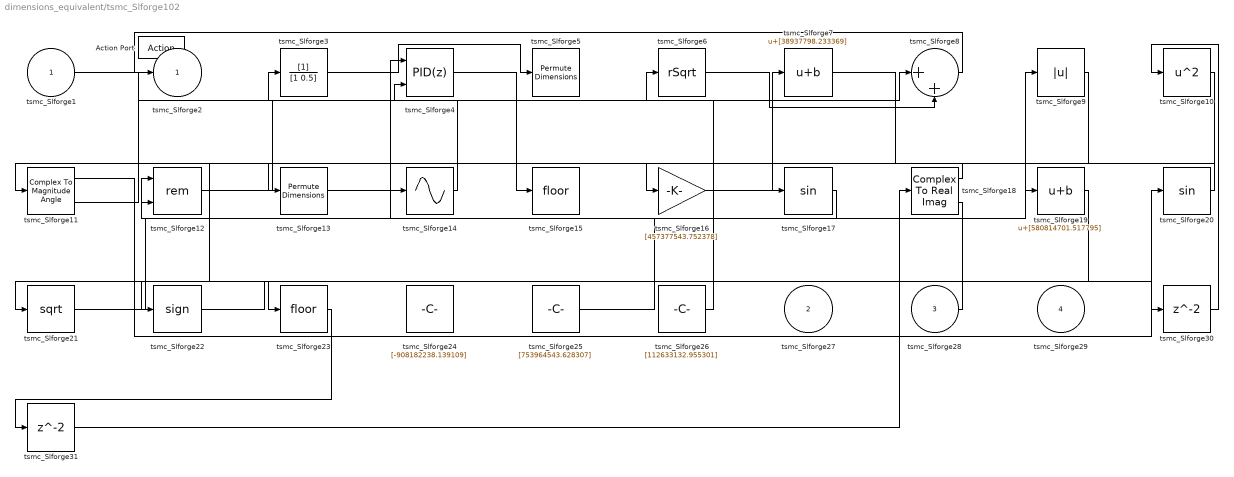
== system dimensions_equivalent/tsmc_Slforge102 ==
  tsmc_Slforge1 : Inport
  tsmc_Slforge27 : Inport  Port=2
  tsmc_Slforge28 : Inport  Port=3
  tsmc_Slforge29 : Inport  Port=4
  Action Port : ActionPort  ActionPortLabel=if { }
  tsmc_Slforge10 : Math  Operator=square  SignedPower=on  SaturateOnIntegerOverflow=on
  tsmc_Slforge11 : ComplexToMagnitudeAngle
  tsmc_Slforge12 : Math  Operator=rem  SignedPower=on  SaturateOnIntegerOverflow=on
  tsmc_Slforge13 : PermuteDimensions
  tsmc_Slforge14 : Sin  TimeSource=Use external signal  SampleTime=0
  tsmc_Slforge15 : Rounding
  tsmc_Slforge16 : Gain  Gain=[457377543.752378]
  tsmc_Slforge17 : Trigonometry
  tsmc_Slforge18 : ComplexToRealImag
  tsmc_Slforge19 : Bias  Bias=[580814701.517795]
  tsmc_Slforge20 : Trigonometry
  tsmc_Slforge21 : Sqrt  SaturateOnIntegerOverflow=on
  tsmc_Slforge22 : Signum
  tsmc_Slforge23 : Rounding
  tsmc_Slforge24 : Constant  Value=[-908182238.139109]  SampleTime=1
  tsmc_Slforge25 : Constant  Value=[753964543.628307]  SampleTime=1
  tsmc_Slforge26 : Constant  Value=[112633132.955301]  SampleTime=1
  tsmc_Slforge3 : DiscreteFilter
  tsmc_Slforge30 : Delay
  tsmc_Slforge31 : Delay
  tsmc_Slforge4 : simulink/Continuous/PID Controller (2DOF)  Controller=PID  TimeDomain=Discrete-time  SampleTime=-1  IntegratorMethod=Forward Euler  FilterMethod=Forward Euler  Form=Parallel  UseFilter=on  ControllerParametersSource=internal  P=1  I=1  D=0  N=100  b=1  c=1  InitialConditionSource=internal  InitialConditionForIntegrator=0  InitialConditionForFilter=0  ExternalReset=none  LimitOutput=off  UpperSaturationLimit=inf  LowerSaturationLimit=-inf  LinearizeAsGain=off  AntiWindupMode=none  Kb=1  TrackingMode=off  Kt=1  PParamMin=[]  PParamMax=[]  IParamMin=[]  IParamMax=[]  DParamMin=[]  DParamMax=[]  NParamMin=[]  NParamMax=[]  bParamMin=[]  bParamMax=[]  cParamMin=[]  cParamMax=[]  KbParamMin=[]  KbParamMax=[]  KtParamMin=[]  KtParamMax=[]  POutMin=[]  POutMax=[]  IOutMin=[]  IOutMax=[]  DOutMin=[]  DOutMax=[]  NOutMin=[]  NOutMax=[]  bOutMin=[]  bOutMax=[]  cOutMin=[]  cOutMax=[]  KbOutMin=[]  KbOutMax=[]  KtOutMin=[]  KtOutMax=[]  IntegratorOutMin=[]  IntegratorOutMax=[]  FilterOutMin=[]  FilterOutMax=[]  SumOutMin=[]  SumOutMax=[]  Sum1OutMin=[]  Sum1OutMax=[]  Sum2OutMin=[]  Sum2OutMax=[]  Sum3OutMin=[]  Sum3OutMax=[]  SumI1OutMin=[]  SumI1OutMax=[]  SumI2OutMin=[]  SumI2OutMax=[]  SumI3OutMin=[]  SumI3OutMax=[]  SumDOutMin=[]  SumDOutMax=[]  SaturationOutMin=[]  SaturationOutMax=[]  IntegratorContinuousStateAttributes=''  IntegratorStateMustResolveToSignalObject=off  IntegratorRTWStateStorageClass=Auto  FilterContinuousStateAttributes=''  FilterStateMustResolveToSignalObject=off  FilterRTWStateStorageClass=Auto  DifferentiatorICPrevScaledInput=0  DifferentiatorOutMin=[]  DifferentiatorOutMax=[]  FilterDiffOutCoefMin=[]  FilterDiffOutCoefMax=[]  SumDenOutMin=[]  SumDenOutMax=[]  SumNumOutMin=[]  SumNumOutMax=[]  ReciprocalOutMin=[]  ReciprocalOutMax=[]  DivideOutMin=[]  DivideOutMax=[]  TunerSelectOption=Transfer Function Based (PID Tuner App)
  tsmc_Slforge5 : PermuteDimensions
  tsmc_Slforge6 : Sqrt  Operator=rSqrt  AlgorithmType=Newton-Raphson  SaturateOnIntegerOverflow=on
  tsmc_Slforge7 : Bias  Bias=[38937798.233369]
  tsmc_Slforge8 : Sum  Inputs=|++
  tsmc_Slforge9 : Abs
  tsmc_Slforge2 : Outport  VectorParamsAs1DForOutWhenUnconnected=off
  wires:
  tsmc_Slforge28/1 -> tsmc_Slforge12/1
  tsmc_Slforge20/1 -> tsmc_Slforge16/1
  tsmc_Slforge25/1 -> tsmc_Slforge9/1
  tsmc_Slforge18/1 -> tsmc_Slforge11/1
  tsmc_Slforge3/1 -> tsmc_Slforge5/1
  tsmc_Slforge14/1 -> tsmc_Slforge3/1
  tsmc_Slforge12/1 -> tsmc_Slforge8/1
  tsmc_Slforge7/1 -> tsmc_Slforge19/1
  tsmc_Slforge8/1 -> tsmc_Slforge2/1
  tsmc_Slforge13/1 -> tsmc_Slforge14/1
  tsmc_Slforge18/2 -> tsmc_Slforge23/1
  tsmc_Slforge16/1 -> tsmc_Slforge7/1
  tsmc_Slforge17/1 -> tsmc_Slforge12/2
  tsmc_Slforge1/1 -> tsmc_Slforge17/1
  tsmc_Slforge11/1 -> tsmc_Slforge20/1
  tsmc_Slforge6/1 -> tsmc_Slforge8/2
  tsmc_Slforge4/1 -> tsmc_Slforge15/1
  tsmc_Slforge19/1 -> tsmc_Slforge21/1
  tsmc_Slforge21/1 -> tsmc_Slforge4/1
  tsmc_Slforge26/1 -> tsmc_Slforge6/1
  tsmc_Slforge11/2 -> tsmc_Slforge4/2
  tsmc_Slforge10/1 -> tsmc_Slforge22/1
  tsmc_Slforge9/1 -> tsmc_Slforge13/1
  tsmc_Slforge22/1 -> tsmc_Slforge30/1
  tsmc_Slforge30/1 -> tsmc_Slforge10/1
  tsmc_Slforge23/1 -> tsmc_Slforge31/1
  tsmc_Slforge31/1 -> tsmc_Slforge18/1

== system dimensions_equivalent/tsmc_Slforge103 ==
  tsmc_Slforge1 : Inport
  tsmc_Slforge26 : Inport  Port=2
  tsmc_Slforge27 : Inport  Port=3
  Action Port : ActionPort  ActionPortLabel=else { }
  tsmc_Slforge10 : Product
  tsmc_Slforge11 : Sin  TimeSource=Use external signal  SampleTime=0
  tsmc_Slforge12 : Sum  Inputs=+-
  tsmc_Slforge13 : Rounding
  tsmc_Slforge14 : PermuteDimensions
  tsmc_Slforge15 : Product  Inputs=*
  tsmc_Slforge16 : MinMax  Function=max
  tsmc_Slforge17 : Assignment  DiagnosticForDimensions=Warning  IndexOptions=Index vector (dialog)  Indices=1  OutputSizes=1
  tsmc_Slforge18 : ComplexToRealImag
  tsmc_Slforge19 : Signum
  tsmc_Slforge20 : Trigonometry
  tsmc_Slforge21 : Math  Operator=log10  SignedPower=on  SaturateOnIntegerOverflow=on
  tsmc_Slforge22 : Sum  Inputs=--
  tsmc_Slforge23 : Sum  Inputs=+-
  tsmc_Slforge24 : Sum  Inputs=+-
  tsmc_Slforge25 : Constant  Value=[803857343.460681]  SampleTime=1
  tsmc_Slforge28 : Delay
  tsmc_Slforge29 : Delay
  tsmc_Slforge3 : Delay
  tsmc_Slforge4 : DiscreteStateSpace  SampleTime=-1
  tsmc_Slforge5 : DiscreteFilter
  tsmc_Slforge6 : simulink/Discrete/Transfer Fcn First Order  PoleZ=0.95  ICPrevOutput=0.0  DoSatur=off
  tsmc_Slforge7 : Sin  TimeSource=Use external signal  SampleTime=0
  tsmc_Slforge8 : PermuteDimensions
  tsmc_Slforge9 : Gain  Gain=[-816431654.639215]
  tsmc_Slforge2 : Outport  VectorParamsAs1DForOutWhenUnconnected=off
  wires:
  tsmc_Slforge4/1 -> tsmc_Slforge17/1, tsmc_Slforge23/2
  tsmc_Slforge6/1 -> tsmc_Slforge12/1
  tsmc_Slforge1/1 -> tsmc_Slforge19/1
  tsmc_Slforge25/1 -> tsmc_Slforge6/1
  tsmc_Slforge15/1 -> tsmc_Slforge5/1
  tsmc_Slforge13/1 -> tsmc_Slforge24/1
  tsmc_Slforge21/1 -> tsmc_Slforge14/1
  tsmc_Slforge11/1 -> tsmc_Slforge18/1
  tsmc_Slforge18/1 -> tsmc_Slforge3/1
  tsmc_Slforge23/1 -> tsmc_Slforge21/1
  tsmc_Slforge8/1 -> tsmc_Slforge7/1
  tsmc_Slforge12/1 -> tsmc_Slforge10/1
  tsmc_Slforge14/1 -> tsmc_Slforge9/1
  tsmc_Slforge3/1 -> tsmc_Slforge17/2
  tsmc_Slforge24/1 -> tsmc_Slforge15/1
  tsmc_Slforge20/1 -> tsmc_Slforge10/2
  tsmc_Slforge10/1 -> tsmc_Slforge8/1
  tsmc_Slforge17/1 -> tsmc_Slforge16/1
  tsmc_Slforge18/2 -> tsmc_Slforge20/1
  tsmc_Slforge5/1 -> tsmc_Slforge2/1
  tsmc_Slforge19/1 -> tsmc_Slforge22/1
  tsmc_Slforge22/1 -> tsmc_Slforge11/1
  tsmc_Slforge26/1 -> tsmc_Slforge23/1, tsmc_Slforge12/2
  tsmc_Slforge7/1 -> tsmc_Slforge13/1
  tsmc_Slforge27/1 -> tsmc_Slforge24/2
  tsmc_Slforge16/1 -> tsmc_Slforge28/1
  tsmc_Slforge28/1 -> tsmc_Slforge22/2
  tsmc_Slforge9/1 -> tsmc_Slforge29/1
  tsmc_Slforge29/1 -> tsmc_Slforge4/1

== system dimensions_equivalent/tsmc_Slforge104 ==
  tsmc_Slforge1 : Inport
  tsmc_Slforge27 : Inport  Port=2
  tsmc_Slforge28 : Inport  Port=3
  Action Port : ActionPort  ActionPortLabel=if { }
  tsmc_Slforge10 : Squeeze
  tsmc_Slforge11 : Sum  Inputs=+-
  tsmc_Slforge12 : Product  Inputs=**
  tsmc_Slforge13 : Product  Inputs=*
  tsmc_Slforge14 : MinMax  Inputs=3
  tsmc_Slforge15 : Product  Inputs=*
  tsmc_Slforge16 : UnaryMinus
  tsmc_Slforge17 : Trigonometry
  tsmc_Slforge18 : Sin  TimeSource=Use external signal  SampleTime=0
  tsmc_Slforge19 : Trigonometry
  tsmc_Slforge20 : UnaryMinus
  tsmc_Slforge21 : ComplexToRealImag
  tsmc_Slforge22 : Product  Inputs=**
  tsmc_Slforge23 : ComplexToMagnitudeAngle
  tsmc_Slforge24 : Bias  Bias=[471750109.876930]
  tsmc_Slforge25 : Squeeze
  tsmc_Slforge26 : Constant  Value=[328866239.654391]  SampleTime=1
  tsmc_Slforge29 : Delay
  tsmc_Slforge3 : DiscreteStateSpace  SampleTime=-1
  tsmc_Slforge30 : Delay
  tsmc_Slforge4 : DiscreteFir
  tsmc_Slforge5 : DiscreteFir
  tsmc_Slforge6 : Reshape
  tsmc_Slforge7 : Reshape
  tsmc_Slforge8 : Product  Inputs=*
  tsmc_Slforge9 : simulink/Math Operations/Slider Gain  gain=1  low=0  high=2
  tsmc_Slforge2 : Outport  VectorParamsAs1DForOutWhenUnconnected=off
  wires:
  tsmc_Slforge10/1 -> tsmc_Slforge16/1
  tsmc_Slforge14/1 -> tsmc_Slforge5/1
  tsmc_Slforge3/1 -> tsmc_Slforge25/1
  tsmc_Slforge13/1 -> tsmc_Slforge10/1
  tsmc_Slforge11/1 -> tsmc_Slforge6/1
  tsmc_Slforge8/1 -> tsmc_Slforge3/1
  tsmc_Slforge15/1 -> tsmc_Slforge9/1
  tsmc_Slforge18/1 -> tsmc_Slforge17/1
  tsmc_Slforge20/1 -> tsmc_Slforge12/1
  tsmc_Slforge19/1 -> tsmc_Slforge22/1
  tsmc_Slforge4/1 -> tsmc_Slforge8/1
  tsmc_Slforge26/1 -> tsmc_Slforge22/2
  tsmc_Slforge21/1 -> tsmc_Slforge18/1
  tsmc_Slforge17/1 -> tsmc_Slforge23/1
  tsmc_Slforge25/1 -> tsmc_Slforge14/1
  tsmc_Slforge1/1 -> tsmc_Slforge4/1
  tsmc_Slforge9/1 -> tsmc_Slforge13/1
  tsmc_Slforge22/1 -> tsmc_Slforge11/1
  tsmc_Slforge7/1 -> tsmc_Slforge15/1
  tsmc_Slforge5/1 -> tsmc_Slforge11/2
  tsmc_Slforge28/1 -> tsmc_Slforge12/2
  tsmc_Slforge24/1 -> tsmc_Slforge20/1
  tsmc_Slforge27/1 -> tsmc_Slforge24/1
  tsmc_Slforge12/1 -> tsmc_Slforge21/1
  tsmc_Slforge23/1 -> tsmc_Slforge14/3
  tsmc_Slforge21/2 -> tsmc_Slforge19/1
  tsmc_Slforge23/2 -> tsmc_Slforge2/1
  tsmc_Slforge6/1 -> tsmc_Slforge29/1
  tsmc_Slforge29/1 -> tsmc_Slforge14/2
  tsmc_Slforge16/1 -> tsmc_Slforge30/1
  tsmc_Slforge30/1 -> tsmc_Slforge7/1

== system dimensions_equivalent/tsmc_Slforge105 ==
  tsmc_Slforge1 : Inport
  tsmc_Slforge24 : Inport  Port=2
  tsmc_Slforge25 : Inport  Port=3
  Action Port : ActionPort  ActionPortLabel=else { }
  tsmc_Slforge10 : UnaryMinus
  tsmc_Slforge11 : Abs
  tsmc_Slforge12 : ComplexToMagnitudeAngle
  tsmc_Slforge13 : simulink/Math Operations/MinMax Running Resettable  Function=min  vinit=0.0
  tsmc_Slforge14 : Abs
  tsmc_Slforge15 : Gain  Gain=[-434110884.143707]
  tsmc_Slforge16 : Sum  Inputs=+-
  tsmc_Slforge17 : DotProduct  InputSameDT=on  OutDataTypeStr=Inherit: Inherit via internal rule
  tsmc_Slforge18 : Product  Inputs=**
  tsmc_Slforge19 : Sum  Inputs=|++
  tsmc_Slforge20 : DotProduct  InputSameDT=on  OutDataTypeStr=Inherit: Inherit via internal rule
  tsmc_Slforge21 : Trigonometry
  tsmc_Slforge22 : ComplexToMagnitudeAngle
  tsmc_Slforge23 : Trigonometry
  tsmc_Slforge{26..29} (4 alike) : Delay
  tsmc_Slforge3 : DiscreteFir
  tsmc_Slforge4 : simulink/Discrete/Transfer Fcn Lead or Lag  PoleZ=0.95  ZeroZ=0.75  ICPrevOutput=0.0  ICPrevInput=0.0  DoSatur=off
      settings: SourceProductBaseCode=SL
  tsmc_Slforge5 : Rounding
  tsmc_Slforge6 : Trigonometry
  tsmc_Slforge7 : Sin  TimeSource=Use external signal  SampleTime=0
  tsmc_Slforge8 : Sum  Inputs=+
  tsmc_Slforge9 : Sqrt  SaturateOnIntegerOverflow=on
  tsmc_Slforge2 : Outport  VectorParamsAs1DForOutWhenUnconnected=off
  wires:
  tsmc_Slforge18/1 -> tsmc_Slforge11/1
  tsmc_Slforge10/1 -> tsmc_Slforge14/1
  tsmc_Slforge1/1 -> tsmc_Slforge5/1
  tsmc_Slforge22/1 -> tsmc_Slforge15/1
  tsmc_Slforge15/1 -> tsmc_Slforge18/1
  tsmc_Slforge25/1 -> tsmc_Slforge22/1
  tsmc_Slforge12/1 -> tsmc_Slforge16/1
  tsmc_Slforge13/1 -> tsmc_Slforge21/1
  tsmc_Slforge11/1 -> tsmc_Slforge16/2
  tsmc_Slforge4/1 -> tsmc_Slforge23/1
  tsmc_Slforge8/1 -> tsmc_Slforge12/1
  tsmc_Slforge6/1 -> tsmc_Slforge18/2, tsmc_Slforge7/1
  tsmc_Slforge3/1 -> tsmc_Slforge8/1, tsmc_Slforge19/2
  tsmc_Slforge7/1 -> tsmc_Slforge4/1
  tsmc_Slforge22/2 -> tsmc_Slforge20/1
  tsmc_Slforge23/1 -> tsmc_Slforge13/1
  tsmc_Slforge24/1 -> tsmc_Slforge20/2
  tsmc_Slforge12/2 -> tsmc_Slforge6/1
  tsmc_Slforge17/1 -> tsmc_Slforge19/1
  tsmc_Slforge20/1 -> tsmc_Slforge2/1
  tsmc_Slforge5/1 -> tsmc_Slforge17/1
  tsmc_Slforge9/1 -> tsmc_Slforge10/1
  tsmc_Slforge19/1 -> tsmc_Slforge26/1
  tsmc_Slforge26/1 -> tsmc_Slforge17/2
  tsmc_Slforge16/1 -> tsmc_Slforge27/1
  tsmc_Slforge27/1 -> tsmc_Slforge3/1
  tsmc_Slforge21/1 -> tsmc_Slforge28/1
  tsmc_Slforge28/1 -> tsmc_Slforge13/2
  tsmc_Slforge14/1 -> tsmc_Slforge29/1
  tsmc_Slforge29/1 -> tsmc_Slforge9/1

== system dimensions_equivalent/tsmc_Slforge106 ==
  tsmc_Slforge1 : Inport
  tsmc_Slforge19 : Inport  Port=2
  tsmc_Slforge20 : Inport  Port=3
  tsmc_Slforge21 : Inport  Port=4
  Action Port : ActionPort  ActionPortLabel=if { }
  tsmc_Slforge10 : Product  Inputs=**
  tsmc_Slforge11 : Sum  Inputs=|++
  tsmc_Slforge12 : Sum  Inputs=-+
  tsmc_Slforge13 : MinMax
  tsmc_Slforge14 : Sin  TimeSource=Use external signal  SampleTime=0
  tsmc_Slforge15 : Sum  Inputs=|++
  tsmc_Slforge16 : Constant  Value=[513793503.182090]  SampleTime=1
  tsmc_Slforge17 : Constant  Value=[948875065.565698]  SampleTime=1
  tsmc_Slforge18 : Constant  Value=[547454489.929457]  SampleTime=1
  tsmc_Slforge3 : simulink/Continuous/PID Controller  Controller=PID  TimeDomain=Discrete-time  SampleTime=-1  IntegratorMethod=Forward Euler  FilterMethod=Forward Euler  Form=Parallel  UseFilter=on  ControllerParametersSource=internal  P=1  I=1  D=0  N=100  InitialConditionSource=internal  InitialConditionForIntegrator=0  InitialConditionForFilter=0  ExternalReset=none  LimitOutput=off  UpperSaturationLimit=inf  LowerSaturationLimit=-inf  LinearizeAsGain=off  AntiWindupMode=none  Kb=1  TrackingMode=off  Kt=1  PParamMin=[]  PParamMax=[]  IParamMin=[]  IParamMax=[]  DParamMin=[]  DParamMax=[]  NParamMin=[]  NParamMax=[]  KbParamMin=[]  KbParamMax=[]  KtParamMin=[]  KtParamMax=[]  POutMin=[]  POutMax=[]  IOutMin=[]  IOutMax=[]  DOutMin=[]  DOutMax=[]  NOutMin=[]  NOutMax=[]  KbOutMin=[]  KbOutMax=[]  KtOutMin=[]  KtOutMax=[]  IntegratorOutMin=[]  IntegratorOutMax=[]  FilterOutMin=[]  FilterOutMax=[]  SumOutMin=[]  SumOutMax=[]  SumI1OutMin=[]  SumI1OutMax=[]  SumI2OutMin=[]  SumI2OutMax=[]  SumI3OutMin=[]  SumI3OutMax=[]  SumDOutMin=[]  SumDOutMax=[]  SaturationOutMin=[]  SaturationOutMax=[]  IntegratorContinuousStateAttributes=''  IntegratorStateMustResolveToSignalObject=off  IntegratorRTWStateStorageClass=Auto  FilterContinuousStateAttributes=''  FilterStateMustResolveToSignalObject=off  FilterRTWStateStorageClass=Auto  DifferentiatorICPrevScaledInput=0  DifferentiatorOutMin=[]  DifferentiatorOutMax=[]  FilterDiffOutCoefMin=[]  FilterDiffOutCoefMax=[]  SumDenOutMin=[]  SumDenOutMax=[]  SumNumOutMin=[]  SumNumOutMax=[]  ReciprocalOutMin=[]  ReciprocalOutMax=[]  DivideOutMin=[]  DivideOutMax=[]  TunerSelectOption=Transfer Function Based (PID Tuner App)
  tsmc_Slforge4 : DiscreteTransferFcn
  tsmc_Slforge5 : UnitDelay  SampleTime=-1  HasFrameUpgradeWarning=on
  tsmc_Slforge6 : Squeeze
  tsmc_Slforge7 : UnaryMinus
  tsmc_Slforge8 : Sin  TimeSource=Use external signal  SampleTime=0
  tsmc_Slforge9 : ComplexToMagnitudeAngle
  tsmc_Slforge2 : Outport  VectorParamsAs1DForOutWhenUnconnected=off
  tsmc_Slforge22 : Outport  Port=2  VectorParamsAs1DForOutWhenUnconnected=off
  wires:
  tsmc_Slforge21/1 -> tsmc_Slforge15/1
  tsmc_Slforge15/1 -> tsmc_Slforge13/1
  tsmc_Slforge16/1 -> tsmc_Slforge4/1
  tsmc_Slforge10/1 -> tsmc_Slforge12/1
  tsmc_Slforge4/1 -> tsmc_Slforge22/1
  tsmc_Slforge5/1 -> tsmc_Slforge15/2
  tsmc_Slforge12/1 -> tsmc_Slforge5/1
  tsmc_Slforge13/1 -> tsmc_Slforge9/1
  tsmc_Slforge14/1 -> tsmc_Slforge11/1
  tsmc_Slforge8/1 -> tsmc_Slforge3/1
  tsmc_Slforge17/1 -> tsmc_Slforge11/2
  tsmc_Slforge7/1 -> tsmc_Slforge10/1
  tsmc_Slforge1/1 -> tsmc_Slforge12/2
  tsmc_Slforge3/1 -> tsmc_Slforge10/2
  tsmc_Slforge9/1 -> tsmc_Slforge14/1
  tsmc_Slforge20/1 -> tsmc_Slforge8/1
  tsmc_Slforge9/2 -> tsmc_Slforge2/1
  tsmc_Slforge19/1 -> tsmc_Slforge7/1
  tsmc_Slforge18/1 -> tsmc_Slforge6/1

== system dimensions_equivalent/tsmc_Slforge107 ==
  tsmc_Slforge1 : Inport
  tsmc_Slforge26 : Inport  Port=2
  tsmc_Slforge27 : Inport  Port=3
  Action Port : ActionPort  ActionPortLabel=else { }
  tsmc_Slforge10 : Rounding
  tsmc_Slforge11 : Rounding
  tsmc_Slforge12 : Signum
  tsmc_Slforge13 : MinMax
  tsmc_Slforge14 : Product  Inputs=*
  tsmc_Slforge15 : simulink/Math Operations/MinMax Running Resettable  Function=min  vinit=0.0
  tsmc_Slforge16 : MinMax  Function=max  Inputs=3
  tsmc_Slforge17 : Sqrt  Operator=rSqrt  AlgorithmType=Newton-Raphson  SaturateOnIntegerOverflow=on
  tsmc_Slforge18 : ComplexToRealImag
  tsmc_Slforge19 : Polyval  Coefs=[ +2.081618890e-019, -1.441693666e-014, +4.719686976e-010, -8.536869453e-006, +1.621573104e-001, -8.087801117e+001 ]
  tsmc_Slforge20 : Product
  tsmc_Slforge21 : Gain  Gain=[-396150231.679020]
  tsmc_Slforge22 : Constant  Value=[-270196089.218416]  SampleTime=1
  tsmc_Slforge23 : Constant  Value=[-775229093.544479]  SampleTime=1
  tsmc_Slforge24 : Constant  Value=[-413126145.957520]  SampleTime=1
  tsmc_Slforge25 : Constant  Value=[369157296.296194]  SampleTime=1
  tsmc_Slforge29 : Delay
  tsmc_Slforge3 : DiscreteZeroPole  Poles=[0 0.5]  Gain=1  SampleTime=-1
  tsmc_Slforge4 : Delay
  tsmc_Slforge5 : simulink/Discrete/Transfer Fcn Real Zero  ZeroZ=0.75  ICPrevInput=0.0  DoSatur=off
      settings: SourceProductBaseCode=SL
  tsmc_Slforge6 : Sum  Inputs=+-
  tsmc_Slforge7 : Assignment  DiagnosticForDimensions=Warning  IndexOptions=Index vector (dialog)  Indices=1  OutputSizes=1
  tsmc_Slforge8 : UnaryMinus
  tsmc_Slforge9 : Signum
  tsmc_Slforge2 : Outport  VectorParamsAs1DForOutWhenUnconnected=off
  tsmc_Slforge28 : Outport  Port=2  VectorParamsAs1DForOutWhenUnconnected=off
  wires:
  tsmc_Slforge18/1 -> tsmc_Slforge7/1
  tsmc_Slforge9/1 -> tsmc_Slforge28/1
  tsmc_Slforge21/1 -> tsmc_Slforge4/1
  tsmc_Slforge6/1 -> tsmc_Slforge7/2
  tsmc_Slforge25/1 -> tsmc_Slforge14/1
  tsmc_Slforge14/1 -> tsmc_Slforge5/1
  tsmc_Slforge20/1 -> tsmc_Slforge13/1
  tsmc_Slforge11/1 -> tsmc_Slforge10/1
  tsmc_Slforge10/1 -> tsmc_Slforge15/1
  tsmc_Slforge22/1 -> tsmc_Slforge21/1
  tsmc_Slforge7/1 -> tsmc_Slforge16/1
  tsmc_Slforge13/1 -> tsmc_Slforge15/2
  tsmc_Slforge3/1 -> tsmc_Slforge20/1
  tsmc_Slforge18/2 -> tsmc_Slforge9/1
  tsmc_Slforge8/1 -> tsmc_Slforge3/1
  tsmc_Slforge4/1 -> tsmc_Slforge17/1
  tsmc_Slforge15/1 -> tsmc_Slforge19/1
  tsmc_Slforge27/1 -> tsmc_Slforge16/2
  tsmc_Slforge17/1 -> tsmc_Slforge16/3
  tsmc_Slforge23/1 -> tsmc_Slforge20/2
  tsmc_Slforge12/1 -> tsmc_Slforge6/2
  tsmc_Slforge1/1 -> tsmc_Slforge12/1
  tsmc_Slforge26/1 -> tsmc_Slforge11/1
  tsmc_Slforge24/1 -> tsmc_Slforge2/1
  tsmc_Slforge19/1 -> tsmc_Slforge18/1
  tsmc_Slforge5/1 -> tsmc_Slforge8/1
  tsmc_Slforge16/1 -> tsmc_Slforge29/1
  tsmc_Slforge29/1 -> tsmc_Slforge6/1

== system dimensions_equivalent/tsmc_Slforge52 ==
  tsmc_Slforge1 : Inport
  tsmc_Slforge8 : Inport  Port=2
  tsmc_Slforge9 : Inport  Port=3
  tsmc_Slforge10 : Inport  Port=4
  tsmc_Slforge3 : DiscreteFir  SampleTime=1
  tsmc_Slforge4 : Abs
  tsmc_Slforge5 : MinMax  Function=max  Inputs=2
  tsmc_Slforge6 : Trigonometry
  tsmc_Slforge7 : Constant  Value=[-458811386.285586]  SampleTime=1
  tsmc_Slforge2 : Outport  VectorParamsAs1DForOutWhenUnconnected=off
  wires:
  tsmc_Slforge10/1 -> tsmc_Slforge3/1
  tsmc_Slforge8/1 -> tsmc_Slforge6/1
  tsmc_Slforge6/1 -> tsmc_Slforge4/1
  tsmc_Slforge7/1 -> tsmc_Slforge5/1
  tsmc_Slforge3/1 -> tsmc_Slforge5/2
  tsmc_Slforge1/1 -> tsmc_Slforge2/1
